simulink model "discreto"  (R2020a)
settings: Solver=VariableStepAuto  StartTime=0.0  StopTime=5  RelTol=1e-3
undefined symbols (not defined in the file): T
settings Model: Creator=a1  LastModifiedBy=a1

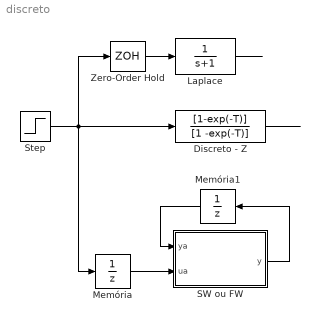
== system discreto ==
  " Laplace" : TransferFcn  Denominator=[1 1]
  Discreto - Z : DiscreteTransferFcn  Numerator=[1-exp(-T)]  Denominator=[1 -exp(-T)]  SampleTime=T
  Memória : UnitDelay  SampleTime=-1  HasFrameUpgradeWarning=on
  Memória1 : UnitDelay  SampleTime=-1  HasFrameUpgradeWarning=on
  SW ou FW : MATLAB Function  TreatAsAtomicUnit=on
  Step : Step  SampleTime=0
  Zero-Order Hold : ZeroOrderHold  SampleTime=T
  wires:
  Step/1 -> Memória/1, Zero-Order Hold/1, Discreto - Z/1
  " Laplace"/1 -> ?
  Discreto - Z/1 -> ?
  Zero-Order Hold/1 -> " Laplace"/1
  Memória/1 -> SW ou FW/2(ua)
  SW ou FW/1(y) -> Memória1/1
  Memória1/1 -> SW ou FW/1(ya)

== matlab function discreto/SW ou FW ==
  data: ya input; y output; ua input
function y = software(ya,ua)

% ya = y(n-1)
% ua = u(n-1)


y = 0.9048*ya + 0.0952*ua;
